simulink model "pd_gravity_comp"  (R2021a)
settings: Solver=VariableStepAuto  StartTime=0.0  StopTime=10.0  RelTol=1e-3
values from neighbouring files (symbols this model uses):
  Kd = 10    [pd_gravity_comp_script.m]
  Kp = 50    [pd_gravity_comp_script.m]
libraries: roblocks x3
settings Model: Creator=root  LastModifiedBy=root

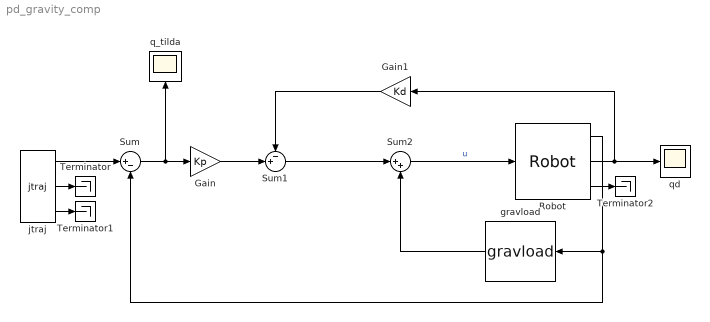
== system pd_gravity_comp ==
  Gain : Gain  Gain=Kp
  Gain1 : Gain  Gain=Kd
  Robot : roblocks/Arm/Robot  robot=ur5  q0=[0 0 0 0 0 0]
  Sum : Sum  Inputs=|+-
  Sum1 : Sum  Inputs=-+|
  Sum2 : Sum  Inputs=|++
  Terminator : Terminator
  Terminator1 : Terminator
  Terminator2 : Terminator
  gravload : roblocks/Arm/gravload  robot=ur5
  jtraj : roblocks/Toolbox/jtraj  q0=[0 0 0 0 0 0]  qf=[pi/4 pi/2 -pi/2 0 0 0]  tmax=10  ts=0.02
  q_tilda : Scope
  qd : Scope
  wires:
  Robot/2 -> qd/1, Gain1/1
  jtraj/1 -> Sum/1
  Robot/1 -> gravload/1, Sum/2
  Gain1/1 -> Sum1/1
  Sum1/1 -> Sum2/1
  Sum2/1 -> Robot/1  "u"
  gravload/1 -> Sum2/2
  Sum/1 -> q_tilda/1, Gain/1
  Gain/1 -> Sum1/2
  jtraj/2 -> Terminator/1
  jtraj/3 -> Terminator1/1
  Robot/3 -> Terminator2/1
